simulink model "bang_bang"  (R2025b)
settings: Solver=FixedStepAuto  StartTime=0.0  StopTime=10.0  FixedStep=0.01  RelTol=1e-3
settings Model: Creator=Junch  LastModifiedBy=11568

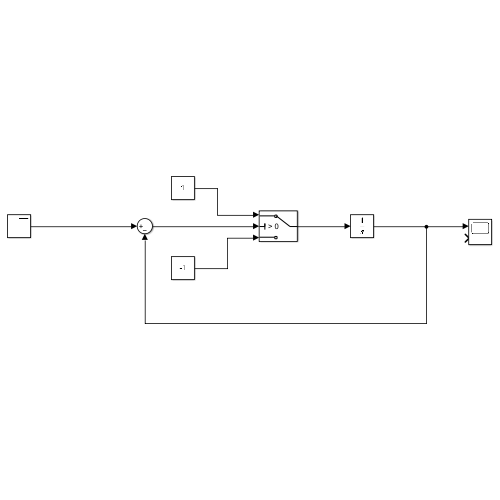
[thumbnail: Simulink's stored preview of the top-level diagram]
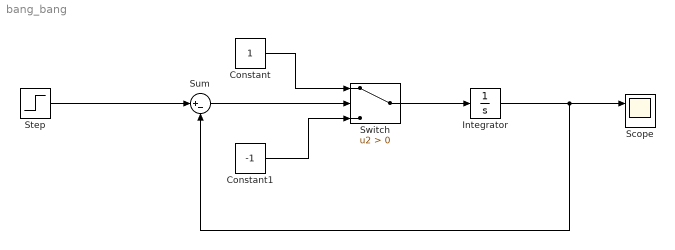
== system bang_bang ==
  Constant : Constant
  Constant1 : Constant  Value=-1
  Integrator : Integrator
  Scope : Scope  NumInputPorts=2
      settings: ActiveDisplayYMinimum=-1.4049954757830743  ActiveDisplayYMaximum=3.1001969562066249
  Step : Step  SampleTime=0
  Sum : Sum  Inputs=|+-
  Switch : Switch  Criteria=u2 > Threshold  SaturateOnIntegerOverflow=off  InputSameDT=off
  wires:
  Integrator/1 -> Sum/2, Scope/1
  Sum/1 -> Switch/2
  Step/1 -> Sum/1
  Switch/1 -> Integrator/1
  Constant/1 -> Switch/1
  Constant1/1 -> Switch/3
